simulink library "csc_eom_six_dof_integration_lib"  (R2014b)
settings: Solver=ode45  StartTime=0.0  StopTime=10.0  RelTol=1e-3
undefined symbols (not defined in the file): int_integrator_rk4
libraries: util_info_lib x3, csu_rrd_rotational_dynamics_lib x2, csu_rrk_rotational_kinematics_lib x2, csu_rtd_translational_dynamics_lib x2, csc_eom_six_dof_integration_lib x2, csu_rtk_translational_kinematics_lib x1
settings Model: Creator=escrane  LastModifiedBy=mstewart

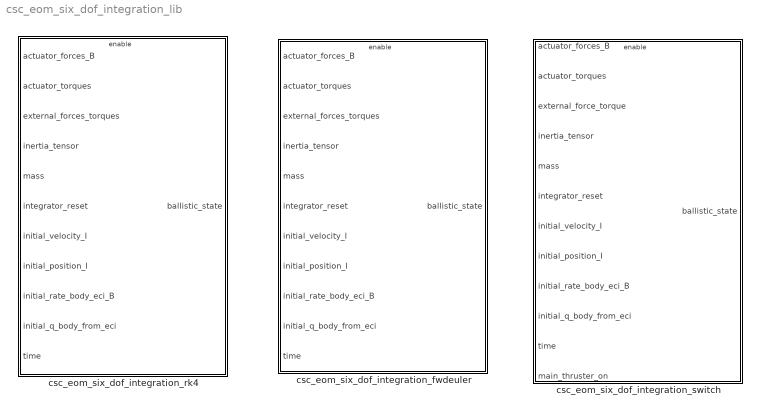
== system csc_eom_six_dof_integration_lib ==
  csc_eom_six_dof_integration_fwdeuler : Subsystem
  csc_eom_six_dof_integration_rk4 : Subsystem
  csc_eom_six_dof_integration_switch : Subsystem

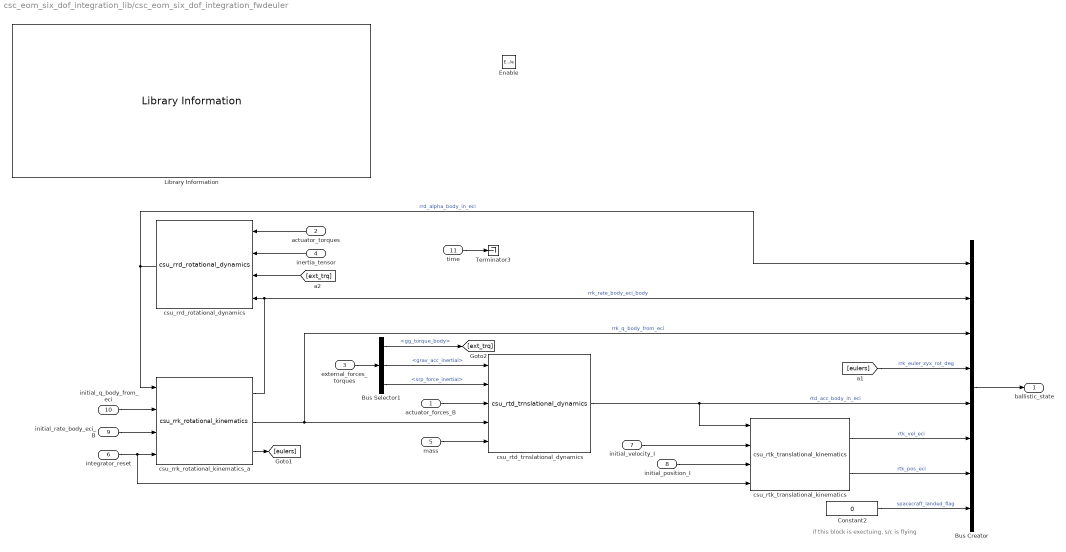
== system csc_eom_six_dof_integration_lib/csc_eom_six_dof_integration_fwdeuler ==
  note: if this block is exectuing, s/c is flying
  actuator_forces_B : Inport
  actuator_torques : Inport  Port=2
  external_forces_torques : Inport  Port=3
  inertia_tensor : Inport  Port=4
  mass : Inport  Port=5
  integrator_reset : Inport  Port=6
  initial_velocity_I : Inport  Port=7
  initial_position_I : Inport  Port=8
  initial_rate_body_eci_B : Inport  Port=9
  initial_q_body_from_eci : Inport  Port=10
  time : Inport  Port=11
  Enable : EnablePort  StatesWhenEnabling=reset
  Bus Creator : BusCreator  Inputs=8  OutDataTypeStr=Bus: lander_state_bus_t
  Bus Selector1 : BusSelector  OutputSignals=gg_torque_body,grav_acc_inertial,srp_force_inertial
  Constant2 : Constant  Value=0
  Library Information : util_info_lib/Library Information  owner='escrane'
  Terminator3 : Terminator
  csu_rrd_rotational_dynamics : csu_rrd_rotational_dynamics_lib/csu_rrd_rotational_dynamics
  csu_rrk_rotational_kinematics_a : csu_rrk_rotational_kinematics_lib/csu_rrk_rotational_kinematics
  csu_rtd_trnslational_dynamics : csu_rtd_translational_dynamics_lib/csu_rtd_trnslational_dynamics
  csu_rtk_translational_kinematics : csu_rtk_translational_kinematics_lib/csu_rtk_translational_kinematics
  ballistic_state : Outport
  wires:
  Constant2/1 -> Bus Creator/8  "spacecraft_landed_flag"
  [ext_trq] -> csu_rrd_rotational_dynamics/3
  Bus Selector1/2 -> csu_rtd_trnslational_dynamics/1  "<grav_acc_inertial>"
  Bus Selector1/1 -> [ext_trq]  "<gg_torque_body>"
  Bus Selector1/3 -> csu_rtd_trnslational_dynamics/2  "<srp_force_inertial>"
  external_forces_torques/1 -> Bus Selector1/1
  Bus Creator/1 -> ballistic_state/1
  csu_rrk_rotational_kinematics_a/2 -> csu_rtd_trnslational_dynamics/4, Bus Creator/3  "rrk_q_body_from_eci"
  csu_rrd_rotational_dynamics/1 -> Bus Creator/1, csu_rrk_rotational_kinematics_a/1  "rrd_alpha_body_in_eci"
  [eulers] -> Bus Creator/4  "rrk_euler_zyx_rot_deg"
  csu_rrk_rotational_kinematics_a/1 -> Bus Creator/2, csu_rrd_rotational_dynamics/4  "rrk_rate_body_eci_body"
  csu_rtd_trnslational_dynamics/1 -> Bus Creator/5, csu_rtk_translational_kinematics/1  "rtd_acc_body_in_eci"
  csu_rtk_translational_kinematics/1 -> Bus Creator/6  "rtk_vel_eci"
  csu_rtk_translational_kinematics/2 -> Bus Creator/7  "rtk_pos_eci"
  csu_rrk_rotational_kinematics_a/3 -> [eulers]
  initial_position_I/1 -> csu_rtk_translational_kinematics/3
  initial_velocity_I/1 -> csu_rtk_translational_kinematics/2
  actuator_forces_B/1 -> csu_rtd_trnslational_dynamics/3
  mass/1 -> csu_rtd_trnslational_dynamics/5
  integrator_reset/1 -> csu_rtk_translational_kinematics/4, csu_rrk_rotational_kinematics_a/4
  initial_rate_body_eci_B/1 -> csu_rrk_rotational_kinematics_a/3
  initial_q_body_from_eci/1 -> csu_rrk_rotational_kinematics_a/2
  inertia_tensor/1 -> csu_rrd_rotational_dynamics/2
  actuator_torques/1 -> csu_rrd_rotational_dynamics/1
  time/1 -> Terminator3/1

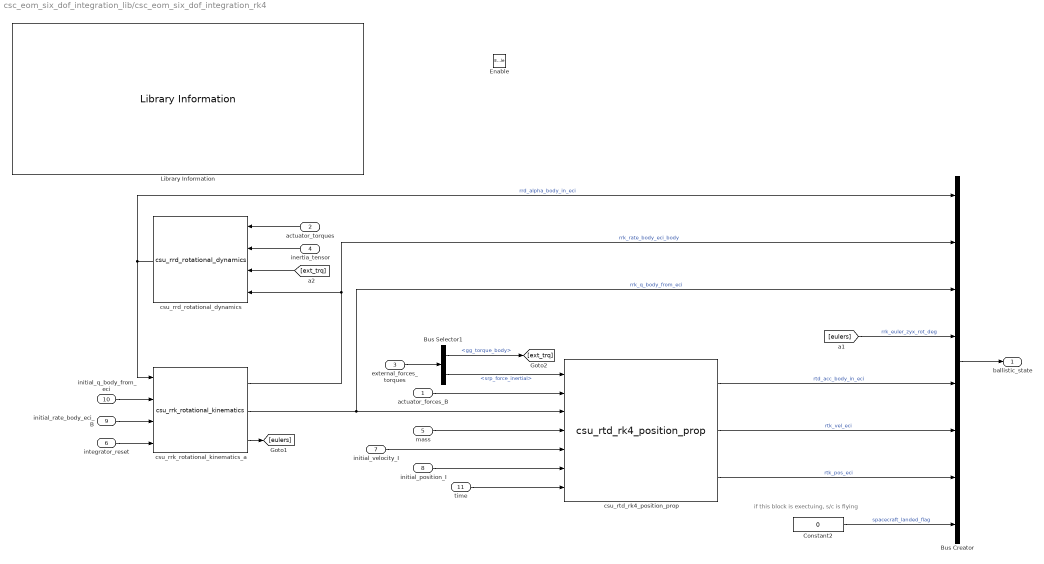
== system csc_eom_six_dof_integration_lib/csc_eom_six_dof_integration_rk4 ==
  note: if this block is exectuing, s/c is flying
  actuator_forces_B : Inport
  actuator_torques : Inport  Port=2
  external_forces_torques : Inport  Port=3
  inertia_tensor : Inport  Port=4
  mass : Inport  Port=5
  integrator_reset : Inport  Port=6
  initial_velocity_I : Inport  Port=7
  initial_position_I : Inport  Port=8
  initial_rate_body_eci_B : Inport  Port=9
  initial_q_body_from_eci : Inport  Port=10
  time : Inport  Port=11
  Enable : EnablePort  StatesWhenEnabling=reset
  Bus Creator : BusCreator  Inputs=8  OutDataTypeStr=Bus: lander_state_bus_t
  Bus Selector1 : BusSelector  OutputSignals=gg_torque_body,srp_force_inertial
  Constant2 : Constant  Value=0
  Library Information : util_info_lib/Library Information  owner='escrane'
  csu_rrd_rotational_dynamics : csu_rrd_rotational_dynamics_lib/csu_rrd_rotational_dynamics
  csu_rrk_rotational_kinematics_a : csu_rrk_rotational_kinematics_lib/csu_rrk_rotational_kinematics
  csu_rtd_rk4_position_prop : csu_rtd_translational_dynamics_lib/csu_rtd_rk4_position_prop
  ballistic_state : Outport
  wires:
  Constant2/1 -> Bus Creator/8  "spacecraft_landed_flag"
  Bus Selector1/1 -> [ext_trq]  "<gg_torque_body>"
  Bus Selector1/2 -> csu_rtd_rk4_position_prop/1  "<srp_force_inertial>"
  [ext_trq] -> csu_rrd_rotational_dynamics/3
  external_forces_torques/1 -> Bus Selector1/1
  actuator_torques/1 -> csu_rrd_rotational_dynamics/1
  inertia_tensor/1 -> csu_rrd_rotational_dynamics/2
  initial_q_body_from_eci/1 -> csu_rrk_rotational_kinematics_a/2
  initial_rate_body_eci_B/1 -> csu_rrk_rotational_kinematics_a/3
  integrator_reset/1 -> csu_rrk_rotational_kinematics_a/4
  mass/1 -> csu_rtd_rk4_position_prop/4
  actuator_forces_B/1 -> csu_rtd_rk4_position_prop/2
  csu_rrk_rotational_kinematics_a/3 -> [eulers]
  csu_rtd_rk4_position_prop/3 -> Bus Creator/7  "rtk_pos_eci"
  csu_rtd_rk4_position_prop/2 -> Bus Creator/6  "rtk_vel_eci"
  csu_rtd_rk4_position_prop/1 -> Bus Creator/5  "rtd_acc_body_in_eci"
  csu_rrk_rotational_kinematics_a/1 -> Bus Creator/2, csu_rrd_rotational_dynamics/4  "rrk_rate_body_eci_body"
  [eulers] -> Bus Creator/4  "rrk_euler_zyx_rot_deg"
  csu_rrd_rotational_dynamics/1 -> csu_rrk_rotational_kinematics_a/1, Bus Creator/1  "rrd_alpha_body_in_eci"
  csu_rrk_rotational_kinematics_a/2 -> csu_rtd_rk4_position_prop/3, Bus Creator/3  "rrk_q_body_from_eci"
  Bus Creator/1 -> ballistic_state/1
  initial_velocity_I/1 -> csu_rtd_rk4_position_prop/5
  initial_position_I/1 -> csu_rtd_rk4_position_prop/6
  time/1 -> csu_rtd_rk4_position_prop/7

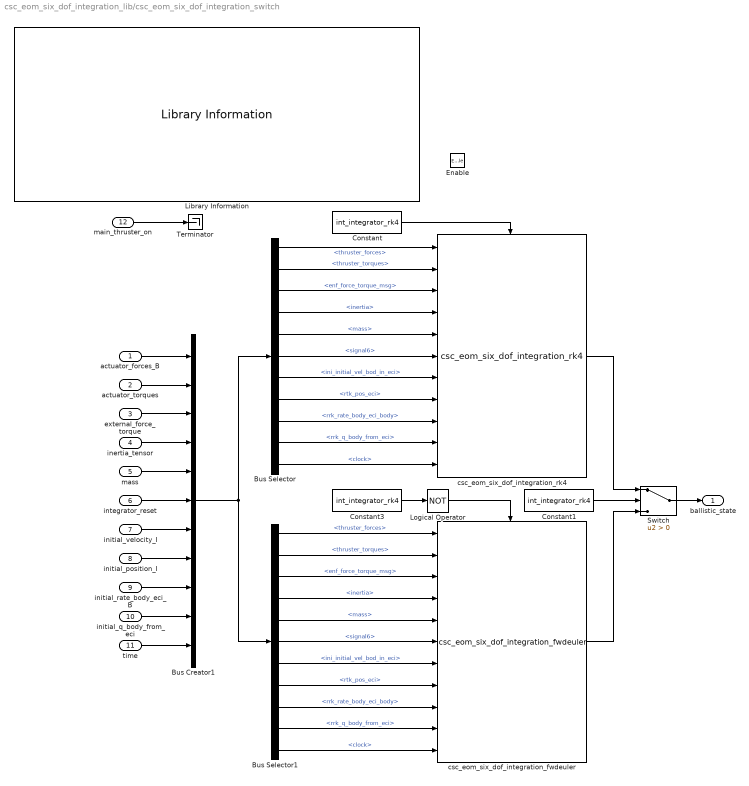
== system csc_eom_six_dof_integration_lib/csc_eom_six_dof_integration_switch ==
  actuator_forces_B : Inport
  actuator_torques : Inport  Port=2
  external_force_torque : Inport  Port=3
  inertia_tensor : Inport  Port=4
  mass : Inport  Port=5
  integrator_reset : Inport  Port=6
  initial_velocity_I : Inport  Port=7
  initial_position_I : Inport  Port=8
  initial_rate_body_eci_B : Inport  Port=9
  initial_q_body_from_eci : Inport  Port=10
  time : Inport  Port=11
  main_thruster_on : Inport  Port=12
  Enable : EnablePort  StatesWhenEnabling=reset
  Bus Creator1 : BusCreator  Inputs=11
  Bus Selector : BusSelector  OutputSignals=thruster_forces,thruster_torques,enf_force_torque_msg,inertia,mass,signal6,ini_initial_vel_bod_in_eci,rtk_pos_eci,rrk_rate_body_eci_body,rrk_q_body_from_eci,clock
  Bus Selector1 : BusSelector  OutputSignals=thruster_forces,thruster_torques,enf_force_torque_msg,inertia,mass,signal6,ini_initial_vel_bod_in_eci,rtk_pos_eci,rrk_rate_body_eci_body,rrk_q_body_from_eci,clock
  Constant : Constant  Value=int_integrator_rk4
  Constant1 : Constant  Value=int_integrator_rk4
  Constant3 : Constant  Value=int_integrator_rk4
  Library Information : util_info_lib/Library Information  owner='escrane'
  Logical Operator : Logic  Operator=NOT  AllPortsSameDT=off  OutDataTypeStr=boolean
  Switch : Switch  Criteria=u2 > Threshold  ZeroCross=off
  Terminator : Terminator
  csc_eom_six_dof_integration_fwdeuler : csc_eom_six_dof_integration_lib/csc_eom_six_dof_integration_fwdeuler
  csc_eom_six_dof_integration_rk4 : csc_eom_six_dof_integration_lib/csc_eom_six_dof_integration_rk4
  ballistic_state : Outport
  wires:
  Bus Selector1/2 -> csc_eom_six_dof_integration_fwdeuler/2  "<thruster_torques>"
  Bus Selector1/3 -> csc_eom_six_dof_integration_fwdeuler/3  "<enf_force_torque_msg>"
  Bus Selector1/4 -> csc_eom_six_dof_integration_fwdeuler/4  "<inertia>"
  Bus Selector1/5 -> csc_eom_six_dof_integration_fwdeuler/5  "<mass>"
  Bus Selector1/6 -> csc_eom_six_dof_integration_fwdeuler/6  "<signal6>"
  Bus Selector1/7 -> csc_eom_six_dof_integration_fwdeuler/7  "<ini_initial_vel_bod_in_eci>"
  Bus Selector1/8 -> csc_eom_six_dof_integration_fwdeuler/8  "<rtk_pos_eci>"
  Bus Selector1/9 -> csc_eom_six_dof_integration_fwdeuler/9  "<rrk_rate_body_eci_body>"
  Bus Selector1/10 -> csc_eom_six_dof_integration_fwdeuler/10  "<rrk_q_body_from_eci>"
  Bus Selector1/11 -> csc_eom_six_dof_integration_fwdeuler/11  "<clock>"
  Bus Selector1/1 -> csc_eom_six_dof_integration_fwdeuler/1  "<thruster_forces>"
  Switch/1 -> ballistic_state/1
  csc_eom_six_dof_integration_fwdeuler/1 -> Switch/3
  csc_eom_six_dof_integration_rk4/1 -> Switch/1
  Bus Creator1/1 -> Bus Selector/1, Bus Selector1/1
  Bus Selector/2 -> csc_eom_six_dof_integration_rk4/2  "<thruster_torques>"
  Bus Selector/3 -> csc_eom_six_dof_integration_rk4/3  "<enf_force_torque_msg>"
  Bus Selector/4 -> csc_eom_six_dof_integration_rk4/4  "<inertia>"
  Bus Selector/5 -> csc_eom_six_dof_integration_rk4/5  "<mass>"
  Bus Selector/6 -> csc_eom_six_dof_integration_rk4/6  "<signal6>"
  Bus Selector/7 -> csc_eom_six_dof_integration_rk4/7  "<ini_initial_vel_bod_in_eci>"
  Bus Selector/8 -> csc_eom_six_dof_integration_rk4/8  "<rtk_pos_eci>"
  Bus Selector/9 -> csc_eom_six_dof_integration_rk4/9  "<rrk_rate_body_eci_body>"
  Bus Selector/10 -> csc_eom_six_dof_integration_rk4/10  "<rrk_q_body_from_eci>"
  Bus Selector/11 -> csc_eom_six_dof_integration_rk4/11  "<clock>"
  Bus Selector/1 -> csc_eom_six_dof_integration_rk4/1  "<thruster_forces>"
  Constant/1 -> csc_eom_six_dof_integration_rk4/Enable
  main_thruster_on/1 -> Terminator/1
  time/1 -> Bus Creator1/11
  initial_q_body_from_eci/1 -> Bus Creator1/10
  initial_rate_body_eci_B/1 -> Bus Creator1/9
  initial_position_I/1 -> Bus Creator1/8
  initial_velocity_I/1 -> Bus Creator1/7
  integrator_reset/1 -> Bus Creator1/6
  mass/1 -> Bus Creator1/5
  inertia_tensor/1 -> Bus Creator1/4
  external_force_torque/1 -> Bus Creator1/3
  actuator_torques/1 -> Bus Creator1/2
  actuator_forces_B/1 -> Bus Creator1/1
  Constant3/1 -> Logical Operator/1
  Logical Operator/1 -> csc_eom_six_dof_integration_fwdeuler/Enable
  Constant1/1 -> Switch/2
